simulink model "simulacionConB"  (R2015a)
settings: Solver=ode45  StartTime=0.0  StopTime=5  MaxStep=0.01  RelTol=1e-3
undefined symbols (not defined in the file or in its folder): tau_init
settings Model: Creator=leinad  LastModifiedBy=leinad
settings SolverCC: ZeroCrossControl=EnableAll  AutoInsertRateTranBlk=on
settings DataIOCC: LimitDataPoints=off  SignalLogging=off  DSMLogging=off

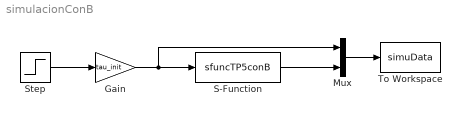
== system simulacionConB ==
  Gain : Gain  Gain=tau_init
  Mux : Mux  Inputs=2
  S-Function : S-Function  FunctionName=sfuncTP5conB  Parameters=[0.2,2,9.8,0.006, -0.05, 0],[0,0]
  Step : Step  SampleTime=0
  To Workspace : ToWorkspace  VariableName=simuData  SaveFormat=Timeseries  SampleTime=-1
  wires:
  Gain/1 -> Mux/1, S-Function/1
  S-Function/1 -> Mux/2
  Mux/1 -> To Workspace/1
  Step/1 -> Gain/1
